simulink model "Simulink_Deliverable_With_Rate_Modulation"  (R2020a)
settings: Solver=FixedStepAuto  StartTime=0.0  StopTime=10.0  FixedStep=1e-3  RelTol=1e-3  EnableMultiTasking=on
undefined symbols (not defined in the file or in its folder): A0, A1, D0, D1, D10, D11, D12, D13, D2, D3, D4, D5, D6, D7, D8, D9, magnitude, PTA0, PTA1, PTA2, PTB2, PTB23, PTB3, PTB9, PTC16, PTC17, PTC2, PTC3, PTC4, PTD0, PTD1, PTD2, PTD3
libraries: frdmk64flib x22, etargetslib x4, dspstat3 x1
settings Model: ExtModeTrigDuration=5  Creator=shivr  LastModifiedBy=aidan_pohqfzv
settings OptimizationCC: EnhancedBackFolding=on  PassReuseOutputArgsAs=Individual arguments  ZeroExternalMemoryAtStartup=off  ZeroInternalMemoryAtStartup=off  MaxStackSize=64  OptimizeBlockOrder=speed  DifferentSizesBufferReuse=on  OptimizationCustomize=off  EfficientTunableParamExpr=on
settings DebuggingCC: ParameterTunabilityLossMsg=error
settings HardwareCC: ProdBitPerPointer=32  ProdBitPerSizeT=32  ProdBitPerPtrDiffT=32  ProdLargestAtomicInteger=Long  ProdLargestAtomicFloat=Double  ProdWordSize=32  ProdHWDeviceType=ARM Compatible->ARM Cortex
settings SFSimCC: MATLABDynamicMemAlloc=off
settings RTWCC: SystemTargetFile=ert.tlc  HardwareBoard=NXP FRDM-K64F  TemplateMakefile=ert_default_tmf  Toolchain=GNU Tools for ARM Embedded Processors
settings CodeAppCC: ForceParamTrailComments=on  IgnoreCustomStorageClasses=off  OperatorAnnotations=on  SimulinkDataObjDesc=on  SFDataObjDesc=on  InsertBlockDesc=on

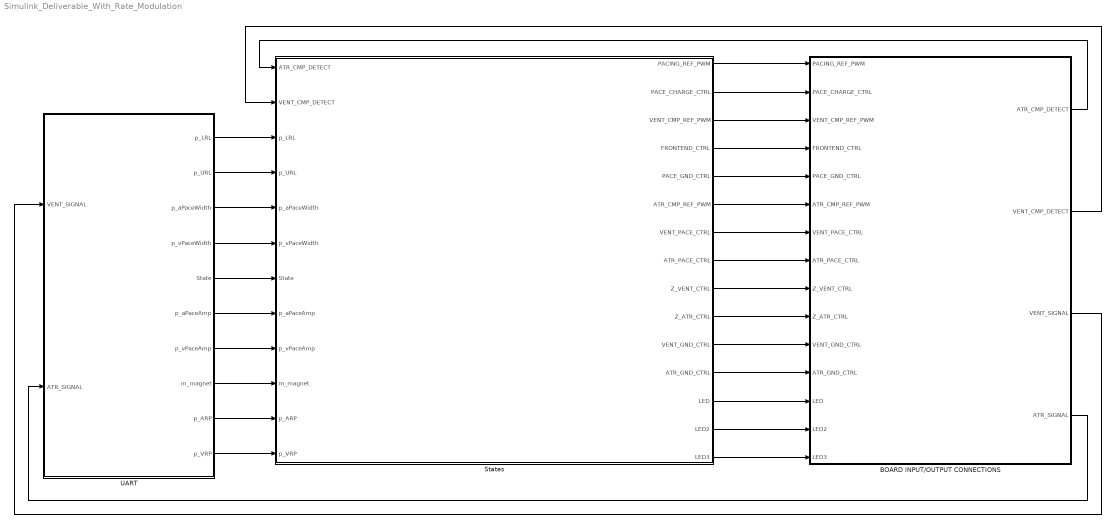
== system Simulink_Deliverable_With_Rate_Modulation ==
  BOARD INPUT/OUTPUT CONNECTIONS : Subsystem
  States : Subsystem
  UART : Subsystem
  wires:
  States/12(ATR_GND_CTRL) -> BOARD INPUT/OUTPUT CONNECTIONS/12(ATR_GND_CTRL)
  States/5(PACE_GND_CTRL) -> BOARD INPUT/OUTPUT CONNECTIONS/5(PACE_GND_CTRL)
  States/11(VENT_GND_CTRL) -> BOARD INPUT/OUTPUT CONNECTIONS/11(VENT_GND_CTRL)
  States/7(VENT_PACE_CTRL) -> BOARD INPUT/OUTPUT CONNECTIONS/7(VENT_PACE_CTRL)
  States/8(ATR_PACE_CTRL) -> BOARD INPUT/OUTPUT CONNECTIONS/8(ATR_PACE_CTRL)
  States/9(Z_VENT_CTRL) -> BOARD INPUT/OUTPUT CONNECTIONS/9(Z_VENT_CTRL)
  States/10(Z_ATR_CTRL) -> BOARD INPUT/OUTPUT CONNECTIONS/10(Z_ATR_CTRL)
  States/4(FRONTEND_CTRL) -> BOARD INPUT/OUTPUT CONNECTIONS/4(FRONTEND_CTRL)
  States/2(PACE_CHARGE_CTRL) -> BOARD INPUT/OUTPUT CONNECTIONS/2(PACE_CHARGE_CTRL)
  States/1(PACING_REF_PWM) -> BOARD INPUT/OUTPUT CONNECTIONS/1(PACING_REF_PWM)
  States/13(LED) -> BOARD INPUT/OUTPUT CONNECTIONS/13(LED)
  BOARD INPUT/OUTPUT CONNECTIONS/1(ATR_CMP_DETECT) -> States/1(ATR_CMP_DETECT)
  BOARD INPUT/OUTPUT CONNECTIONS/2(VENT_CMP_DETECT) -> States/2(VENT_CMP_DETECT)
  States/14(LED2) -> BOARD INPUT/OUTPUT CONNECTIONS/14(LED2)
  States/6(ATR_CMP_REF_PWM) -> BOARD INPUT/OUTPUT CONNECTIONS/6(ATR_CMP_REF_PWM)
  UART/9(p_ARP) -> States/11(p_ARP)
  States/15(LED3) -> BOARD INPUT/OUTPUT CONNECTIONS/15(LED3)
  States/3(VENT_CMP_REF_PWM) -> BOARD INPUT/OUTPUT CONNECTIONS/3(VENT_CMP_REF_PWM)
  UART/10(p_VRP) -> States/12(p_VRP)
  UART/5(State) -> States/7(State)
  UART/1(p_LRL) -> States/3(p_LRL)
  UART/2(p_URL) -> States/4(p_URL)
  UART/3(p_aPaceWidth) -> States/5(p_aPaceWidth)
  UART/4(p_vPaceWidth) -> States/6(p_vPaceWidth)
  UART/6(p_aPaceAmp) -> States/8(p_aPaceAmp)
  UART/7(p_vPaceAmp) -> States/9(p_vPaceAmp)
  UART/8(m_magnet) -> States/10(m_magnet)
  BOARD INPUT/OUTPUT CONNECTIONS/3(VENT_SIGNAL) -> UART/1(VENT_SIGNAL)
  BOARD INPUT/OUTPUT CONNECTIONS/4(ATR_SIGNAL) -> UART/2(ATR_SIGNAL)

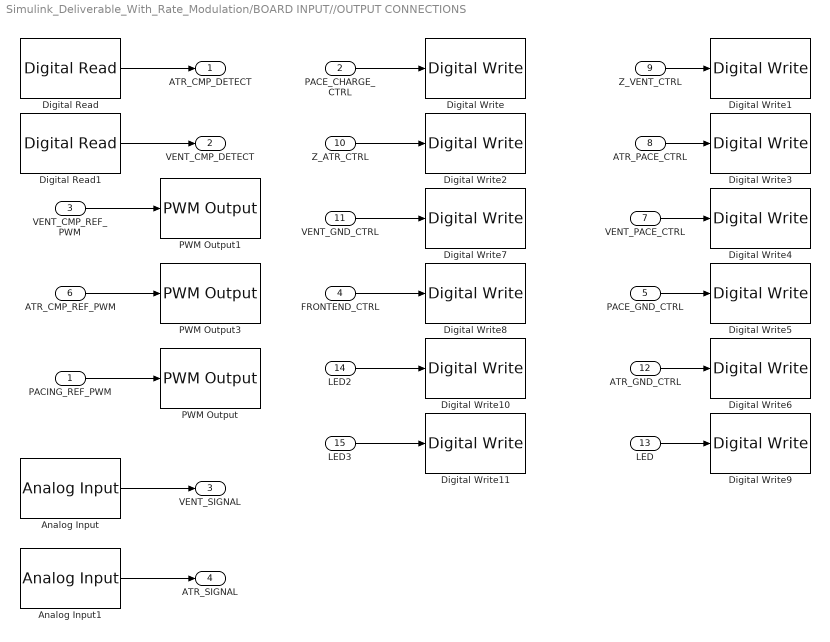
== system Simulink_Deliverable_With_Rate_Modulation/BOARD INPUT//OUTPUT CONNECTIONS ==
  PACING_REF_PWM : Inport
  PACE_CHARGE_CTRL : Inport  Port=2
  VENT_CMP_REF_PWM : Inport  Port=3
  FRONTEND_CTRL : Inport  Port=4
  PACE_GND_CTRL : Inport  Port=5
  ATR_CMP_REF_PWM : Inport  Port=6
  VENT_PACE_CTRL : Inport  Port=7
  ATR_PACE_CTRL : Inport  Port=8
  Z_VENT_CTRL : Inport  Port=9
  Z_ATR_CTRL : Inport  Port=10
  VENT_GND_CTRL : Inport  Port=11
  ATR_GND_CTRL : Inport  Port=12
  LED : Inport  Port=13
  LED2 : Inport  Port=14
  LED3 : Inport  Port=15
  Analog Input : frdmk64flib/Analog Input  Whichpin=PTB3 (A1)  SampleTime=-1
  Analog Input1 : frdmk64flib/Analog Input  Whichpin=PTB2 (A0)  SampleTime=-1
  Digital Read : frdmk64flib/Digital Read  Whichpin=PTC16 (D0)  SampleTime=-1
  Digital Read1 : frdmk64flib/Digital Read  Whichpin=PTC17 (D1)  SampleTime=-1
  Digital Write : frdmk64flib/Digital Write  Whichpin=PTB9 (D2)
  Digital Write1 : frdmk64flib/Digital Write  Whichpin=PTC3 (D7)
  Digital Write10 : frdmk64flib/Digital Write  Whichpin=BLUE_LED
  Digital Write11 : frdmk64flib/Digital Write  Whichpin=GREEN_LED
  Digital Write2 : frdmk64flib/Digital Write  Whichpin=PTB23 (D4)
  Digital Write3 : frdmk64flib/Digital Write  Whichpin=PTA0 (D8)
  Digital Write4 : frdmk64flib/Digital Write  Whichpin=PTC4 (D9)
  Digital Write5 : frdmk64flib/Digital Write  Whichpin=PTD0 (D10)
  Digital Write6 : frdmk64flib/Digital Write  Whichpin=PTD2 (D11)
  Digital Write7 : frdmk64flib/Digital Write  Whichpin=PTD3 (D12)
  Digital Write8 : frdmk64flib/Digital Write  Whichpin=PTD1 (D13)
  Digital Write9 : frdmk64flib/Digital Write  Whichpin=RED_LED
  PWM Output : frdmk64flib/PWM Output  Whichpin=PTA2 (D5)  InitialFrequency=2000  InitialDutyCycle=0
  PWM Output1 : frdmk64flib/PWM Output  Whichpin=PTA1 (D3)  InitialFrequency=2000  InitialDutyCycle=0
  PWM Output3 : frdmk64flib/PWM Output  Whichpin=PTC2 (D6)  InitialFrequency=2000  InitialDutyCycle=100
  ATR_CMP_DETECT : Outport
  VENT_CMP_DETECT : Outport  Port=2
  VENT_SIGNAL : Outport  Port=3
  ATR_SIGNAL : Outport  Port=4
  wires:
  Digital Read/1 -> ATR_CMP_DETECT/1
  Digital Read1/1 -> VENT_CMP_DETECT/1
  VENT_CMP_REF_PWM/1 -> PWM Output1/1
  PACE_CHARGE_CTRL/1 -> Digital Write/1
  Z_ATR_CTRL/1 -> Digital Write2/1
  PACING_REF_PWM/1 -> PWM Output/1
  ATR_CMP_REF_PWM/1 -> PWM Output3/1
  Z_VENT_CTRL/1 -> Digital Write1/1
  ATR_PACE_CTRL/1 -> Digital Write3/1
  VENT_PACE_CTRL/1 -> Digital Write4/1
  PACE_GND_CTRL/1 -> Digital Write5/1
  ATR_GND_CTRL/1 -> Digital Write6/1
  VENT_GND_CTRL/1 -> Digital Write7/1
  FRONTEND_CTRL/1 -> Digital Write8/1
  LED/1 -> Digital Write9/1
  LED2/1 -> Digital Write10/1
  LED3/1 -> Digital Write11/1
  Analog Input1/1 -> ATR_SIGNAL/1
  Analog Input/1 -> VENT_SIGNAL/1

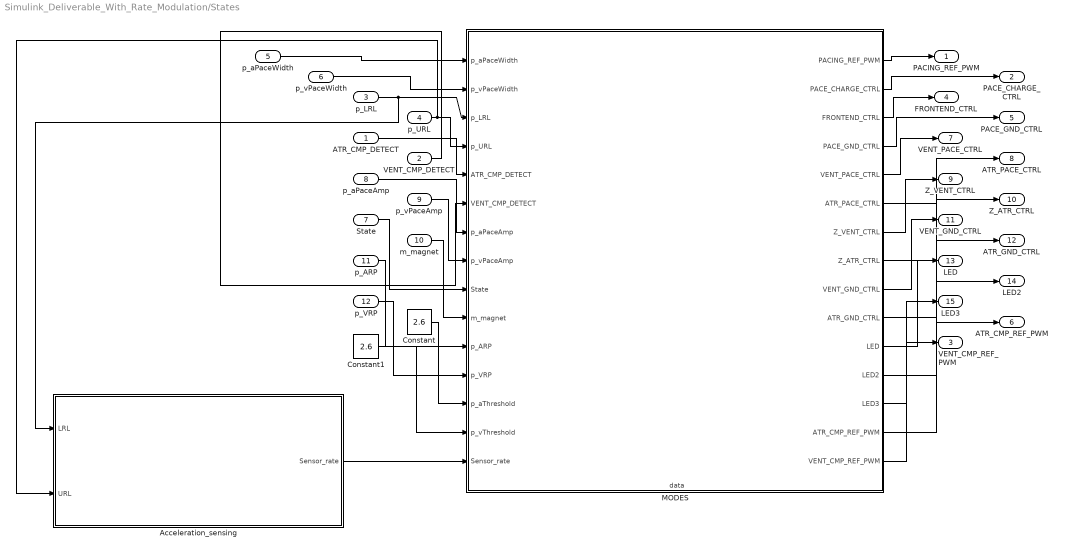
== system Simulink_Deliverable_With_Rate_Modulation/States ==
  ATR_CMP_DETECT : Inport
  VENT_CMP_DETECT : Inport  Port=2
  p_LRL : Inport  Port=3
  p_URL : Inport  Port=4
  p_aPaceWidth : Inport  Port=5
  p_vPaceWidth : Inport  Port=6
  State : Inport  Port=7
  p_aPaceAmp : Inport  Port=8
  p_vPaceAmp : Inport  Port=9
  m_magnet : Inport  Port=10
  p_ARP : Inport  Port=11
  p_VRP : Inport  Port=12
  Acceleration_sensing : Subsystem
  Constant : Constant  Value=2.6
  Constant1 : Constant  Value=2.6
  MODES : Stateflow chart  TreatAsAtomicUnit=on
      settings: PortSchema="{\"entries\":[{\"content\":{\"sides\":[{\"content\":{\"connectorIds\":[\"In1\",\"In2\",\"In3\",\"In4\",\"In5\",\"In6\",\"In7\",\"In8\",\"In9\",\"In10\",\"In11\",\"In12\",\"In13\",\"In14\",\"In15\"]},\"type\":\"ConnectorPlacement.EquallySpacedRectSide\",\"uuid\":\"8502a3c5-6307-4e02-81ee-17e1a35cc298\"},{\"content\":{\"connectorIds\":[\"Out2\",\"Out3\",\"Out4\",\"Out5\",\"Out6\",\"Out7\",\"Out8\",\"Out9\",\"Out10\",\"Out11\",\"Out12\",\"Out15\",\"Out14\",\"Out13\",\"Out16\"],\"side\":\"RIGHT\"},\"type\":\"ConnectorPlacement.EquallySpacedRectSide\",\"uuid\":\"71555ad9-e88e-4949-94fd-af1b739ca2ca\"},{\"content\":{\"connectorIds\":[],\"side\":\"TOP\"},\"type\":\"ConnectorPlacement.EquallySpacedRectSide\",\"uuid\":\"f0239cae-2fc2-4d44-ac00-93735ab3ef8c\"},{\"content\":{\"connectorIds\":[\"Out1\"],\"side\":\"BOTTOM\"},\"type\":\"ConnectorPlacement.EquallySpacedRectSide\",\"uuid\":\"7d1612d5-a202-47d8-98e6-e2ca77499232\"}]},\"type\":\"ConnectorPlacement.EquallySpacedConnector\",\"uuid\":\"0a066545-78b2-4ddc-84c3-90461cea3699\"}],\"packageUris\":[\"http://schema.mathworks.com/mf0/Connector/19700101\"],\"version\":\"1.0\"}"
  PACING_REF_PWM : Outport
  PACE_CHARGE_CTRL : Outport  Port=2
  VENT_CMP_REF_PWM : Outport  Port=3
  FRONTEND_CTRL : Outport  Port=4
  PACE_GND_CTRL : Outport  Port=5
  ATR_CMP_REF_PWM : Outport  Port=6
  VENT_PACE_CTRL : Outport  Port=7
  ATR_PACE_CTRL : Outport  Port=8
  Z_VENT_CTRL : Outport  Port=9
  Z_ATR_CTRL : Outport  Port=10
  VENT_GND_CTRL : Outport  Port=11
  ATR_GND_CTRL : Outport  Port=12
  LED : Outport  Port=13
  LED2 : Outport  Port=14
  LED3 : Outport  Port=15
  wires:
  p_aPaceWidth/1 -> MODES/1(p_aPaceWidth)
  MODES/6(VENT_PACE_CTRL) -> VENT_PACE_CTRL/1
  MODES/4(FRONTEND_CTRL) -> FRONTEND_CTRL/1
  MODES/2(PACING_REF_PWM) -> PACING_REF_PWM/1
  MODES/7(ATR_PACE_CTRL) -> ATR_PACE_CTRL/1
  MODES/8(Z_VENT_CTRL) -> Z_VENT_CTRL/1
  MODES/5(PACE_GND_CTRL) -> PACE_GND_CTRL/1
  MODES/9(Z_ATR_CTRL) -> Z_ATR_CTRL/1
  MODES/3(PACE_CHARGE_CTRL) -> PACE_CHARGE_CTRL/1
  MODES/10(VENT_GND_CTRL) -> VENT_GND_CTRL/1
  MODES/11(ATR_GND_CTRL) -> ATR_GND_CTRL/1
  MODES/12(LED) -> LED/1
  p_LRL/1 -> Acceleration_sensing/1(LRL), MODES/3(p_LRL)
  p_URL/1 -> Acceleration_sensing/2(URL), MODES/4(p_URL)
  ATR_CMP_DETECT/1 -> MODES/5(ATR_CMP_DETECT)
  VENT_CMP_DETECT/1 -> MODES/6(VENT_CMP_DETECT)
  p_aPaceAmp/1 -> MODES/7(p_aPaceAmp)
  m_magnet/1 -> MODES/10(m_magnet)
  MODES/15(LED2) -> LED2/1
  p_vPaceWidth/1 -> MODES/2(p_vPaceWidth)
  p_vPaceAmp/1 -> MODES/8(p_vPaceAmp)
  MODES/13(ATR_CMP_REF_PWM) -> ATR_CMP_REF_PWM/1
  p_ARP/1 -> MODES/11(p_ARP)
  MODES/14(LED3) -> LED3/1
  p_VRP/1 -> MODES/12(p_VRP)
  MODES/16(VENT_CMP_REF_PWM) -> VENT_CMP_REF_PWM/1
  Constant/1 -> MODES/13(p_aThreshold)
  Constant1/1 -> MODES/14(p_vThreshold)
  State/1 -> MODES/9(State)
  Acceleration_sensing/1(Sensor_rate) -> MODES/15(Sensor_rate)

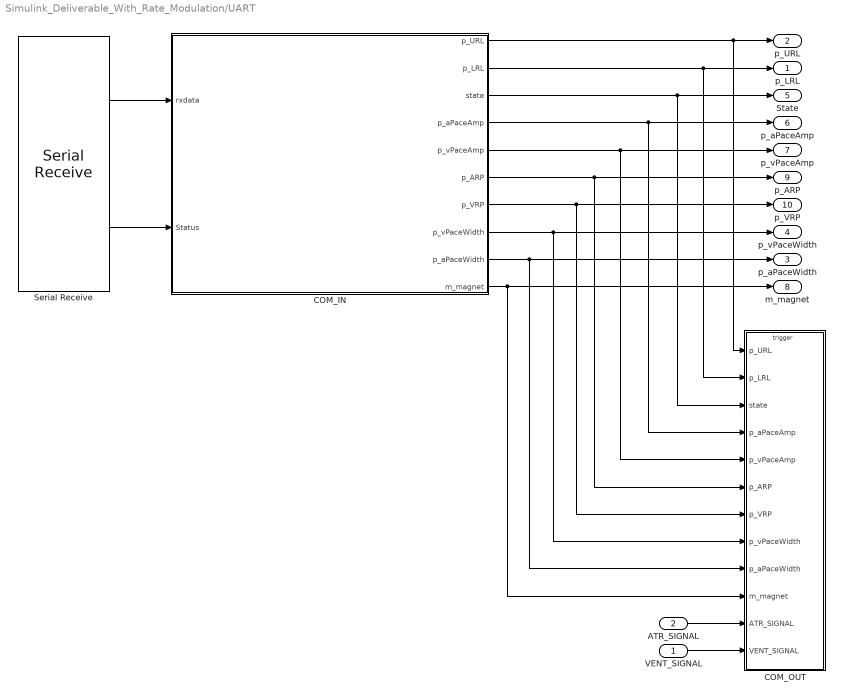
== system Simulink_Deliverable_With_Rate_Modulation/UART ==
  VENT_SIGNAL : Inport
  ATR_SIGNAL : Inport  Port=2
  COM_IN : Stateflow chart  TreatAsAtomicUnit=on
  COM_OUT : Subsystem
  Serial Receive : frdmk64flib/Serial Receive  SCIModule=0  Baudrate=uint32(9600)  Parity=None  StopBits=1  HardwareFlowControl=None  ByteOrder=LittleEndian  DataType=uint8  DataLength=14  BlockingMode=off  OutputStatus=on  SampleTime=-1
  p_LRL : Outport
  p_URL : Outport  Port=2
  p_aPaceWidth : Outport  Port=3
  p_vPaceWidth : Outport  Port=4
  State : Outport  Port=5
  p_aPaceAmp : Outport  Port=6
  p_vPaceAmp : Outport  Port=7
  m_magnet : Outport  Port=8
  p_ARP : Outport  Port=9
  p_VRP : Outport  Port=10
  wires:
  COM_IN/4(p_aPaceAmp) -> p_aPaceAmp/1, COM_OUT/4(p_aPaceAmp)
  COM_IN/6(p_ARP) -> p_ARP/1, COM_OUT/6(p_ARP)
  COM_IN/7(p_VRP) -> p_VRP/1, COM_OUT/7(p_VRP)
  COM_IN/5(p_vPaceAmp) -> p_vPaceAmp/1, COM_OUT/5(p_vPaceAmp)
  COM_IN/1(p_URL) -> p_URL/1, COM_OUT/1(p_URL)
  COM_IN/8(p_vPaceWidth) -> p_vPaceWidth/1, COM_OUT/8(p_vPaceWidth)
  COM_IN/9(p_aPaceWidth) -> p_aPaceWidth/1, COM_OUT/9(p_aPaceWidth)
  COM_IN/2(p_LRL) -> p_LRL/1, COM_OUT/2(p_LRL)
  COM_IN/3(state) -> State/1, COM_OUT/3(state)
  Serial Receive/1 -> COM_IN/1(rxdata)
  Serial Receive/2 -> COM_IN/2(Status)
  COM_IN/10(m_magnet) -> m_magnet/1, COM_OUT/10(m_magnet)
  ATR_SIGNAL/1 -> COM_OUT/11(ATR_SIGNAL)
  VENT_SIGNAL/1 -> COM_OUT/12(VENT_SIGNAL)

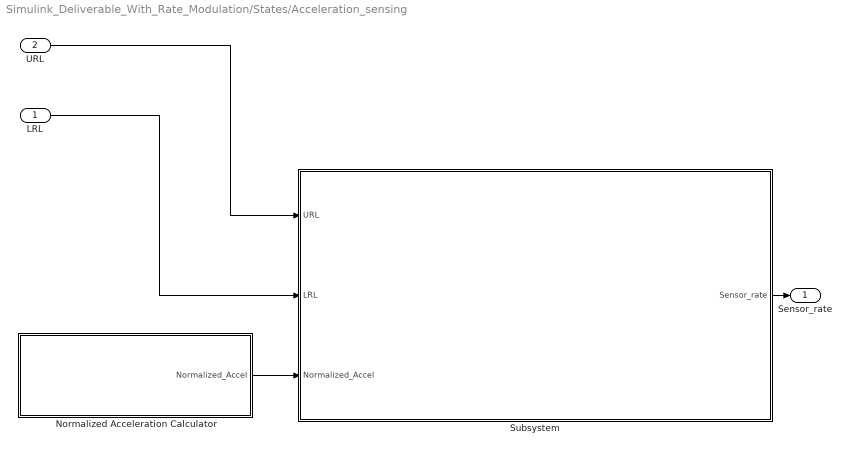
== system Simulink_Deliverable_With_Rate_Modulation/States/Acceleration_sensing ==
  LRL : Inport
  URL : Inport  Port=2
  Normalized Acceleration Calculator : Subsystem
  Subsystem : Subsystem
  Sensor_rate : Outport
  wires:
  Normalized Acceleration Calculator/1(Normalized_Accel) -> Subsystem/3(Normalized_Accel)
  LRL/1 -> Subsystem/2(LRL)
  URL/1 -> Subsystem/1(URL)
  Subsystem/1(Sensor_rate) -> Sensor_rate/1

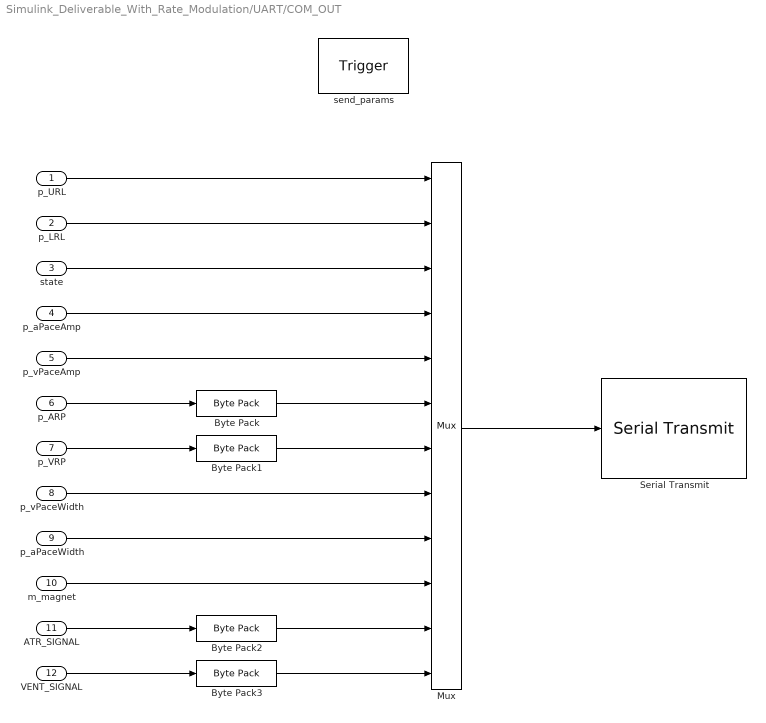
== system Simulink_Deliverable_With_Rate_Modulation/UART/COM_OUT ==
  p_URL : Inport
  p_LRL : Inport  Port=2
  state : Inport  Port=3
  p_aPaceAmp : Inport  Port=4
  p_vPaceAmp : Inport  Port=5
  p_ARP : Inport  Port=6
  p_VRP : Inport  Port=7
  p_vPaceWidth : Inport  Port=8
  p_aPaceWidth : Inport  Port=9
  m_magnet : Inport  Port=10
  ATR_SIGNAL : Inport  Port=11
  VENT_SIGNAL : Inport  Port=12
  send_params : TriggerPort  TriggerType=function-call  IsSimulinkFunction=on  FunctionName=send_params  VariantControl=Variant  PortDimensions=1
  Byte Pack{,1..3} (4 alike) : etargetslib/Byte Pack  datatypes={'double'}  byteAlign=1
  Mux : Mux  Inputs=12
  Serial Transmit : frdmk64flib/Serial Transmit  SCIModule=0  Baudrate=uint32(9600)  Parity=None  StopBits=1  HardwareFlowControl=None  ByteOrder=LittleEndian  BlockingMode=on  OutputStatus=off
  wires:
  p_URL/1 -> Mux/1
  p_LRL/1 -> Mux/2
  state/1 -> Mux/3
  p_aPaceAmp/1 -> Mux/4
  p_vPaceAmp/1 -> Mux/5
  p_ARP/1 -> Byte Pack/1
  Byte Pack/1 -> Mux/6
  p_VRP/1 -> Byte Pack1/1
  Byte Pack1/1 -> Mux/7
  p_vPaceWidth/1 -> Mux/8
  p_aPaceWidth/1 -> Mux/9
  m_magnet/1 -> Mux/10
  ATR_SIGNAL/1 -> Byte Pack2/1
  VENT_SIGNAL/1 -> Byte Pack3/1
  Byte Pack2/1 -> Mux/11
  Byte Pack3/1 -> Mux/12
  Mux/1 -> Serial Transmit/1

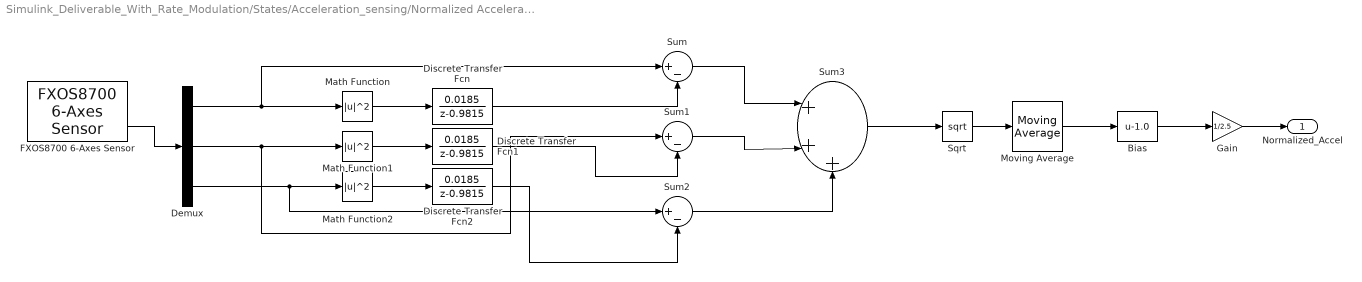
== system Simulink_Deliverable_With_Rate_Modulation/States/Acceleration_sensing/Normalized Acceleration Calculator ==
  Bias : Bias  Bias=-1.0
  Demux : Demux  Outputs=3
  Discrete Transfer Fcn : DiscreteTransferFcn  Numerator=[0.0185]  Denominator=[1 -0.9815]
  Discrete Transfer Fcn1 : DiscreteTransferFcn  Numerator=[0.0185]  Denominator=[1 -0.9815]
  Discrete Transfer Fcn2 : DiscreteTransferFcn  Numerator=[0.0185]  Denominator=[1 -0.9815]
  FXOS8700 6-Axes Sensor : frdmk64flib/FXOS8700 6-Axes Sensor  Activesensor=Accelerometer and Magnetometer  ODR=800Hz  HybridODR=400Hz  Accelfullrange=-4g to +4g  SampleTime=-1
  Gain : Gain  Gain=1/2.5
  Math Function : Math  Operator=magnitude^2  SaturateOnIntegerOverflow=on
  Math Function1 : Math  Operator=magnitude^2  SaturateOnIntegerOverflow=on
  Math Function2 : Math  Operator=magnitude^2  SaturateOnIntegerOverflow=on
  Moving Average : dspstat3/Moving Average  Method=Sliding window  ForgettingFactorPort=off  SpecifyWindowLength=on  WindowLength=10  ForgettingFactor=0.9  SimulateUsing=Code generation
  Sqrt : Sqrt  SaturateOnIntegerOverflow=on
  Sum : Sum  Inputs=|+-
  Sum1 : Sum  Inputs=|+-
  Sum2 : Sum  Inputs=|+-
  Sum3 : Sum  Inputs=|+++
  Normalized_Accel : Outport
  wires:
  Sum/1 -> Sum3/1
  FXOS8700 6-Axes Sensor/2 -> Demux/1
  Demux/2 -> Sum1/1, Math Function1/1
  Demux/3 -> Sum2/1, Math Function2/1
  Discrete Transfer Fcn/1 -> Sum/2
  Math Function1/1 -> Discrete Transfer Fcn1/1
  Math Function/1 -> Discrete Transfer Fcn/1
  Demux/1 -> Sum/1, Math Function/1
  Sum1/1 -> Sum3/2
  Math Function2/1 -> Discrete Transfer Fcn2/1
  Discrete Transfer Fcn2/1 -> Sum2/2
  Sum2/1 -> Sum3/3
  Discrete Transfer Fcn1/1 -> Sum1/2
  Sum3/1 -> Sqrt/1
  Sqrt/1 -> Moving Average/1
  Moving Average/1 -> Bias/1
  Bias/1 -> Gain/1
  Gain/1 -> Normalized_Accel/1

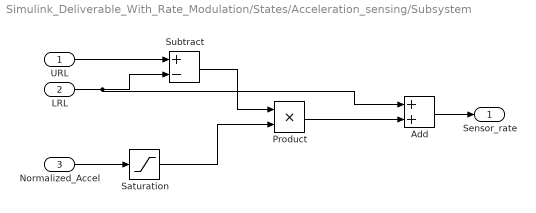
== system Simulink_Deliverable_With_Rate_Modulation/States/Acceleration_sensing/Subsystem ==
  URL : Inport
  LRL : Inport  Port=2
  Normalized_Accel : Inport  Port=3
  Add : Sum
  Product : Product
  Saturation : Saturate  UpperLimit=1  LowerLimit=0
  Subtract : Sum  Inputs=+-
  Sensor_rate : Outport
  wires:
  URL/1 -> Subtract/1
  LRL/1 -> Add/1, Subtract/2
  Subtract/1 -> Product/1
  Product/1 -> Add/2
  Normalized_Accel/1 -> Saturation/1
  Saturation/1 -> Product/2
  Add/1 -> Sensor_rate/1

== stateflow chart Simulink_Deliverable_With_Rate_Modulation/UART/COM_IN ==
  state set_param
    entry:
    p_LRL = rxdata(3);
    p_URL = rxdata(4);
    state = rxdata(5);
    p_aPaceAmp = rxdata(6);
    p_vPaceAmp = rxdata(7);
    p_ARP = typecast(rxdata(8:9), 'uint16');
    p_VRP = typecast(rxdata(10:11), 'uint16');
    p_aPaceWidth = rxdata(12);
    p_vPaceWidth = rxdata(13);
    m_magnet = rxdata(14);
  state Nominal
    entry:
    p_LRL = 120;
    p_URL = 60;
    state = 1;
    p_aPaceAmp = 3.5;
    p_vPaceAmp = 3.5;
    p_ARP = 500;
    p_VRP = 500;
    p_aPaceWidth = 0.4;
    p_vPaceWidth = 0.4;
    m_magnet = 0;
  state Standby
  state echo_param
    entry:
    send_params();
  set_param -> Standby
  (default) -> Nominal
  (junction 9) -> set_param [order 1] : [rxdata(2) == hex2dec ('55')]
  (junction 10) -> Standby [order 2]
  Nominal -> Standby
  Standby -> (junction 10) : [Status == 0]
  (junction 10) -> (junction 9) [order 1] : [rxdata(1)==hex2dec('16')]
  (junction 9) -> echo_param [order 2] : [rxdata(2) == hex2dec ('22')]
  echo_param -> Standby
  data: rxdata input; p_URL output; p_LRL output; Status input; state output; p_aPaceAmp output; p_vPaceAmp output; p_ARP output int16; p_VRP output uint16; p_vPaceWidth output; p_aPaceWidth output; m_magnet output

== stateflow chart Simulink_Deliverable_With_Rate_Modulation/States/MODES ==
  state AOO
    state Prep
      entry:
      FRONTEND_CTRL=false;                              %sensing off
      %start charging C22
      ATR_PACE_CTRL = false;                    %Dont pace Atrium
      VENT_PACE_CTRL = false;         %Vent pacing off in AOO
      %convert pace amp into a duty cycle
      PACING_REF_PWM = p_aPaceAmp/5*100;
      PACE_CHARGE_CTRL = true;   %start charging capacitor
      %discharge blocking (combined state)
      PACE_GND_CTRL = true;    %connect ground to capacitor
      Z_ATR_CTRL= false;        %disable zeroing in atr and vent
      Z_VENT_CTRL=false;
      ATR_GND_CTRL = true;               %connects atrial ground
      VENT_GND_CTRL = false;  %disconnect ventricle ground
      LED = false;                                                 % turn off LED
    state Pace
      entry:
      PACE_CHARGE_CTRL = false;   %stop charging C
      ATR_PACE_CTRL = true;                   %pace atrium
      ATR_GND_CTRL = false;         %disconnect ground
      LED = true;                                   %flash the red led
    (default) -> AOO.Prep
    AOO.Prep -> AOO.Pace : [after(60000/p_LRL-p_aPaceWidth, msec)]
    AOO.Pace -> AOO.Prep : [after(p_aPaceWidth, msec)]
  state VOO
    state VOO_Prep_State
      entry:
      FRONTEND_CTRL=false;                          %sensing off
      %charging
      ATR_PACE_CTRL = false;                 %dont pace atrium
      VENT_PACE_CTRL=false;                   %dont pace vent
      %convert vPaceAmp into duty cycle
      PACING_REF_PWM = p_vPaceAmp/5*100;
      PACE_CHARGE_CTRL=true;                %start charging
      %discharging
      PACE_GND_CTRL=true;             %connect C to ground
      Z_ATR_CTRL = false; %disable zeroing for atr and vent
      Z_VENT_CTRL=false;
      ATR_GND_CTRL = false;    %disconnect atrium ground
      VENT_GND_CTRL=true;      %connect ventricle ground
      LED2 = false;                                 % turn off blue LED
    state VOO_Pace_State
      entry:
      PACE_CHARGE_CTRL=false; %stop charging C
      VENT_GND_CTRL=false; %unground ventricle
      VENT_PACE_CTRL=true; %pace ventricle
      LED2 = true; %turn on blue LED
    (default) -> VOO.VOO_Prep_State
    VOO.VOO_Prep_State -> VOO.VOO_Pace_State : [after(60000.0/p_LRL - p_vPaceWidth,msec)]
    VOO.VOO_Pace_State -> VOO.VOO_Prep_State : [after(p_vPaceWidth,msec)]
  state AAI
    state AAI_CHARGING_DISCHARGING
      entry:
      FRONTEND_CTRL = true; %enable sensing
      %charge capacitor exactly like AOO
      ATR_PACE_CTRL = false;
      PACE_CHARGE_CTRL = true;
      PACE_GND_CTRL = true;
      VENT_PACE_CTRL = false;
      PACING_REF_PWM = p_aPaceAmp/5*100;
      %discharge
      ATR_GND_CTRL = true;
      VENT_PACE_CTRL = false;
      VENT_GND_CTRL = false;
      Z_ATR_CTRL = false;
      Z_VENT_CTRL = false;
      LED3 = false;
      %set the reference comparison PWM
      ATR_CMP_REF_PWM = p_aThreshold/5*100;
    state AAI_PACING
      entry:
      %turn off sensing
      FRONTEND_CTRL = false;
      %Pace like aoo
      PACE_CHARGE_CTRL = false;
      ATR_PACE_CTRL = true;
      ATR_GND_CTRL = false;
      LED3 = true;
    state AAI_REFRACTORY
      entry:
      %enter refractory if natural atrium pulse
      % is detected and wait for p_ARP
      LED2 = ~LED2;
    (default) -> AAI.AAI_CHARGING_DISCHARGING
    AAI.AAI_CHARGING_DISCHARGING -> AAI.AAI_PACING [order 1] : [ATR_CMP_DETECT==false&&after((60000/p_LRL-p_aPaceWidth), msec)]
    AAI.AAI_PACING -> AAI.AAI_CHARGING_DISCHARGING : [after(p_aPaceWidth, msec)]
    AAI.AAI_REFRACTORY -> AAI.AAI_CHARGING_DISCHARGING : [after(p_ARP, msec)]
    AAI.AAI_CHARGING_DISCHARGING -> AAI.AAI_REFRACTORY [order 2] : [ATR_CMP_DETECT == true]
  state state_selector
  state VVI
    state VVI_SENSING
      entry:
      FRONTEND_CTRL = true; %enable sensing
      %charge and discharge exactly like VOO
      ATR_PACE_CTRL = false;
      PACE_CHARGE_CTRL = true;
      PACE_GND_CTRL = true;
      VENT_PACE_CTRL = false;
      PACING_REF_PWM = p_vPaceAmp/5*100;
      %discharge
      ATR_GND_CTRL =false;
      VENT_GND_CTRL = true;
      Z_ATR_CTRL = false;
      Z_VENT_CTRL = false;
      LED3 = false;
      %Set the comparison reference PWM
      VENT_CMP_REF_PWM = p_vThreshold/5*100;
    state VVI_PACING
      entry:
      %turn off sensing
      FRONTEND_CTRL = false;
      %pace like VOO
      PACE_CHARGE_CTRL = false;
      PACE_GND_CTRL = true;
      VENT_PACE_CTRL = true;
      VENT_GND_CTRL = false;
      LED3 = true;
    state VVI_REFRACTORY
      entry:
      %if ventricle pulse is detected:
      %wait p_VRP
      LED2 = ~LED2;
    (default) -> VVI.VVI_SENSING
    VVI.VVI_SENSING -> VVI.VVI_PACING [order 1] : [VENT_CMP_DETECT==false&&after((60000/p_LRL-p_vPaceWidth), msec)]
    VVI.VVI_PACING -> VVI.VVI_SENSING : [after(p_vPaceWidth, msec)]
    VVI.VVI_REFRACTORY -> VVI.VVI_SENSING : [after(p_VRP, msec)]
    VVI.VVI_SENSING -> VVI.VVI_REFRACTORY [order 2] : [VENT_CMP_DETECT == true]
  state AOOR
    state Prep
      entry:
      FRONTEND_CTRL=false;                              %sensing off
      %start charging C22
      ATR_PACE_CTRL = false;                    %Dont pace Atrium
      VENT_PACE_CTRL = false;         %Vent pacing off in AOO
      %convert pace amp into a duty cycle
      PACING_REF_PWM = p_aPaceAmp/5*100;
      PACE_CHARGE_CTRL = true;   %start charging capacitor
      %discharge blocking (combined state)
      PACE_GND_CTRL = true;    %connect ground to capacitor
      Z_ATR_CTRL= false;        %disable zeroing in atr and vent
      Z_VENT_CTRL=false;
      ATR_GND_CTRL = true;               %connects atrial ground
      VENT_GND_CTRL = false;  %disconnect ventricle ground
      LED = false;                                                 % turn off LED
    state Pace
      entry:
      PACE_CHARGE_CTRL = false;   %stop charging C
      ATR_PACE_CTRL = true;                   %pace atrium
      ATR_GND_CTRL = false;         %disconnect ground
      LED = true;                                   %flash the red led
    (default) -> AOOR.Prep
    AOOR.Prep -> AOOR.Pace : [after(60000/Sensor_rate-p_aPaceWidth, msec)]
    AOOR.Pace -> AOOR.Prep : [after(p_aPaceWidth, msec)]
  state VOOR
    state VOO_Prep_State
      entry:
      FRONTEND_CTRL=false;                          %sensing off
      %charging
      ATR_PACE_CTRL = false;                 %dont pace atrium
      VENT_PACE_CTRL=false;                   %dont pace vent
      %convert vPaceAmp into duty cycle
      PACING_REF_PWM = p_vPaceAmp/5*100;
      PACE_CHARGE_CTRL=true;                %start charging
      %discharging
      PACE_GND_CTRL=true;             %connect C to ground
      Z_ATR_CTRL = false; %disable zeroing for atr and vent
      Z_VENT_CTRL=false;
      ATR_GND_CTRL = false;    %disconnect atrium ground
      VENT_GND_CTRL=true;      %connect ventricle ground
      LED2 = false;                                 % turn off blue LED
    state VOO_Pace_State
      entry:
      PACE_CHARGE_CTRL=false; %stop charging C
      VENT_GND_CTRL=false; %unground ventricle
      VENT_PACE_CTRL=true; %pace ventricle
      LED2 = true; %turn on blue LED
    (default) -> VOOR.VOO_Prep_State
    VOOR.VOO_Prep_State -> VOOR.VOO_Pace_State : [after(60000.0/Sensor_rate - p_vPaceWidth,msec)]
    VOOR.VOO_Pace_State -> VOOR.VOO_Prep_State : [after(p_vPaceWidth,msec)]
  state AAIR
    state AAI_CHARGING_DISCHARGING
      entry:
      FRONTEND_CTRL = true; %enable sensing
      %charge capacitor exactly like AOO
      ATR_PACE_CTRL = false;
      PACE_CHARGE_CTRL = true;
      PACE_GND_CTRL = true;
      VENT_PACE_CTRL = false;
      PACING_REF_PWM = p_aPaceAmp/5*100;
      %discharge
      ATR_GND_CTRL = true;
      VENT_PACE_CTRL = false;
      VENT_GND_CTRL = false;
      Z_ATR_CTRL = false;
      Z_VENT_CTRL = false;
      LED3 = false;
      %set the reference comparison PWM
      ATR_CMP_REF_PWM = p_aThreshold/5*100;
    state AAI_PACING
      entry:
      %turn off sensing
      FRONTEND_CTRL = false;
      %Pace like aoo
      PACE_CHARGE_CTRL = false;
      ATR_PACE_CTRL = true;
      ATR_GND_CTRL = false;
      LED3 = true;
    state AAI_REFRACTORY
      entry:
      %enter refractory if natural atrium pulse
      % is detected and wait for p_ARP
      LED2 = ~LED2;
    (default) -> AAIR.AAI_CHARGING_DISCHARGING
    AAIR.AAI_CHARGING_DISCHARGING -> AAIR.AAI_PACING [order 1] : [ATR_CMP_DETECT==false&&after((60000/Sensor_rate-p_aPaceWidth), msec)]
    AAIR.AAI_PACING -> AAIR.AAI_CHARGING_DISCHARGING : [after(p_aPaceWidth, msec)]
    AAIR.AAI_REFRACTORY -> AAIR.AAI_CHARGING_DISCHARGING : [after(p_ARP, msec)]
    AAIR.AAI_CHARGING_DISCHARGING -> AAIR.AAI_REFRACTORY [order 2] : [ATR_CMP_DETECT == true]
  state VVIR
    state VVI_SENSING
      entry:
      FRONTEND_CTRL = true; %enable sensing
      %charge and discharge exactly like VOO
      ATR_PACE_CTRL = false;
      PACE_CHARGE_CTRL = true;
      PACE_GND_CTRL = true;
      VENT_PACE_CTRL = false;
      PACING_REF_PWM = p_vPaceAmp/5*100;
      %discharge
      ATR_GND_CTRL =false;
      VENT_GND_CTRL = true;
      Z_ATR_CTRL = false;
      Z_VENT_CTRL = false;
      LED3 = false;
      %Set the comparison reference PWM
      VENT_CMP_REF_PWM = p_vThreshold/5*100;
    state VVI_PACING
      entry:
      %turn off sensing
      FRONTEND_CTRL = false;
      %pace like VOO
      PACE_CHARGE_CTRL = false;
      PACE_GND_CTRL = true;
      VENT_PACE_CTRL = true;
      VENT_GND_CTRL = false;
      LED3 = true;
    state VVI_REFRACTORY
      entry:
      %if ventricle pulse is detected:
      %wait p_VRP
      LED2 = ~LED2;
    (default) -> VVIR.VVI_SENSING
    VVIR.VVI_SENSING -> VVIR.VVI_PACING [order 1] : [VENT_CMP_DETECT==false&&after((60000/Sensor_rate-p_vPaceWidth), msec)]
    VVIR.VVI_PACING -> VVIR.VVI_SENSING : [after(p_vPaceWidth, msec)]
    VVIR.VVI_REFRACTORY -> VVIR.VVI_SENSING : [after(p_VRP, msec)]
    VVIR.VVI_SENSING -> VVIR.VVI_REFRACTORY [order 2] : [VENT_CMP_DETECT == true]
  state_selector -> AOO [order 1] : [State == 1&&m_magnet==0]
  state_selector -> VOO [order 2] : [m_magnet == 1 || State == 2]
  state_selector -> AAI [order 3] : [State == 3&&m_magnet==0]
  state_selector -> VVI [order 4] : [State == 4&&m_magnet==0]
  (default) -> state_selector
  state_selector -> AOOR [order 8] : [State == 8&&m_magnet==0]
  state_selector -> VOOR [order 7] : [State == 7&&m_magnet==0]
  state_selector -> AAIR [order 5] : [State == 5&&m_magnet==0]
  state_selector -> VVIR [order 6] : [State == 6&&m_magnet==1]
  data: data output; PACING_REF_PWM output; PACE_CHARGE_CTRL output; FRONTEND_CTRL output; PACE_GND_CTRL output; VENT_PACE_CTRL output; ATR_PACE_CTRL output; Z_VENT_CTRL output; Z_ATR_CTRL output; VENT_GND_CTRL output; ATR_GND_CTRL output; LED output; ATR_CMP_REF_PWM output; LED3 output; p_aPaceWidth input; p_vPaceWidth input; p_LRL input; p_URL input; ATR_CMP_DETECT input; VENT_CMP_DETECT input; p_aPaceAmp input; p_vPaceAmp input; State input; m_magnet input; LED2 output; p_ARP input int16; p_VRP input int16; VENT_CMP_REF_PWM output; p_aThreshold input; p_vThreshold input; Sensor_rate input
